simulink model "case4"  (R2024b)
settings: Solver=FixedStepAuto  StartTime=0  StopTime=1  FixedStep=1e-7  RelTol=1e-3
values from neighbouring files (symbols this model uses):
  SG_D_1_D = 0.01056    [IEEE9_case_parameters.m]    (also in case1_parameters.m; case2_parameters.m; case3_parameters.m; case4_parameters.m)
  SG_D_1_EnableSaturation = 0    [IEEE9_case_parameters.m]    (also in case1_parameters.m; case2_parameters.m; case3_parameters.m; case4_parameters.m)
  SG_D_1_f0 = 60    [IEEE9_case_parameters.m]    (also in case1_parameters.m; case2_parameters.m; case3_parameters.m; case4_parameters.m)
  SG_D_1_H = 7.5    [IEEE9_case_parameters.m]    (also in case1_parameters.m; case2_parameters.m; case3_parameters.m; case4_parameters.m)
  SG_D_1_K_A = 20    [IEEE9_case_parameters.m]    (also in case1_parameters.m; case2_parameters.m; case3_parameters.m; case4_parameters.m)
  SG_D_1_K_E = 1.000000e+1    (= 10)    [IEEE9_case_parameters.m]    (also in case1_parameters.m; case2_parameters.m; case3_parameters.m; case4_parameters.m)
  SG_D_1_K_F = 2.363    [IEEE9_case_parameters.m]    (also in case1_parameters.m; case2_parameters.m; case3_parameters.m; case4_parameters.m)
  SG_D_1_K_s = 0.5    [IEEE9_case_parameters.m]    (also in case1_parameters.m = 5; case2_parameters.m = 5; case3_parameters.m = 5; case4_parameters.m = 5)
  SG_D_1_R_a = 0.001088    [IEEE9_case_parameters.m]    (also in case1_parameters.m; case2_parameters.m; case3_parameters.m; case4_parameters.m)
  SG_D_1_S_A = 1    [IEEE9_case_parameters.m]    (also in case1_parameters.m; case2_parameters.m; case3_parameters.m; case4_parameters.m)
  SG_D_1_S_B = 0.103    [IEEE9_case_parameters.m]    (also in case1_parameters.m; case2_parameters.m; case3_parameters.m; case4_parameters.m)
  SG_D_1_S_N = 10.659857    [IEEE9_case_parameters.m]    (also in case1_parameters.m; case2_parameters.m; case3_parameters.m; case4_parameters.m)
  SG_D_1_SpeedPara = 200    [IEEE9_case_parameters.m]    (also in case1_parameters.m; case2_parameters.m; case3_parameters.m; case4_parameters.m)
  SG_D_1_T_0 = 0.720173    [IEEE9_case_parameters.m]    (also in case1_parameters.m = 0.755522; case2_parameters.m = 0.808931; case3_parameters.m = 0.869402; case4_parameters.m = 0.729316)
  SG_D_1_T_1 = 0.3    [IEEE9_case_parameters.m]    (also in case1_parameters.m; case2_parameters.m; case3_parameters.m; case4_parameters.m)
  SG_D_1_T_2 = 0.05    [IEEE9_case_parameters.m]    (also in case1_parameters.m; case2_parameters.m; case3_parameters.m; case4_parameters.m)
  SG_D_1_T_3 = 0.02    [IEEE9_case_parameters.m]    (also in case1_parameters.m; case2_parameters.m; case3_parameters.m; case4_parameters.m)
  SG_D_1_T_4 = 0.005    [IEEE9_case_parameters.m]    (also in case1_parameters.m; case2_parameters.m; case3_parameters.m; case4_parameters.m)
  SG_D_1_T_A = 0.02    [IEEE9_case_parameters.m]    (also in case1_parameters.m; case2_parameters.m; case3_parameters.m; case4_parameters.m)
  SG_D_1_T_dd = 8.000000e+0    (= 8)    [IEEE9_case_parameters.m]    (also in case1_parameters.m; case2_parameters.m; case3_parameters.m; case4_parameters.m)
  SG_D_1_T_ddd = 0.04    [IEEE9_case_parameters.m]    (also in case1_parameters.m; case2_parameters.m; case3_parameters.m; case4_parameters.m)
  SG_D_1_T_E = 0.314    [IEEE9_case_parameters.m]    (also in case1_parameters.m; case2_parameters.m; case3_parameters.m; case4_parameters.m)
  SG_D_1_T_F = 0.35    [IEEE9_case_parameters.m]    (also in case1_parameters.m; case2_parameters.m; case3_parameters.m; case4_parameters.m)
  SG_D_1_T_qd = 0.8    [IEEE9_case_parameters.m]    (also in case1_parameters.m; case2_parameters.m; case3_parameters.m; case4_parameters.m)
  SG_D_1_T_qdd = 0.02    [IEEE9_case_parameters.m]    (also in case1_parameters.m; case2_parameters.m; case3_parameters.m; case4_parameters.m)
  SG_D_1_T_speed = 0.1    [IEEE9_case_parameters.m]    (also in case1_parameters.m = 200; case2_parameters.m = 200; case3_parameters.m = 200; case4_parameters.m = 200)
  SG_D_1_T_w = 0.5    [IEEE9_case_parameters.m]    (also in case1_parameters.m; case2_parameters.m; case3_parameters.m; case4_parameters.m)
  SG_D_1_V_ref = 1.990276    [IEEE9_case_parameters.m]    (also in case1_parameters.m = 2.042296; case2_parameters.m = 2.051388; case3_parameters.m = 2.089584; case4_parameters.m = 2.01845)
  SG_D_1_w_ref = 376.991118    [IEEE9_case_parameters.m]    (also in case1_parameters.m; case2_parameters.m; case3_parameters.m; case4_parameters.m)
  SG_D_1_wb = 6.000000e+1    (= 60)    [IEEE9_case_parameters.m]    (also in case1_parameters.m; case2_parameters.m; case3_parameters.m; case4_parameters.m)
  SG_D_1_x_d = 1.9    [IEEE9_case_parameters.m]    (also in case1_parameters.m; case2_parameters.m; case3_parameters.m; case4_parameters.m)
  SG_D_1_x_dd = 0.302    [IEEE9_case_parameters.m]    (also in case1_parameters.m; case2_parameters.m; case3_parameters.m; case4_parameters.m)
  SG_D_1_x_ddd = 0.204    [IEEE9_case_parameters.m]    (also in case1_parameters.m; case2_parameters.m; case3_parameters.m; case4_parameters.m)
  SG_D_1_x_l = 0.05    [IEEE9_case_parameters.m]    (also in case1_parameters.m; case2_parameters.m; case3_parameters.m; case4_parameters.m)
  SG_D_1_x_q = 1.3    [IEEE9_case_parameters.m]    (also in case1_parameters.m; case2_parameters.m; case3_parameters.m; case4_parameters.m)
  SG_D_1_x_qd = 0.5    [IEEE9_case_parameters.m]    (also in case1_parameters.m; case2_parameters.m; case3_parameters.m; case4_parameters.m)
  SG_D_1_x_qdd = 0.3    [IEEE9_case_parameters.m]    (also in case1_parameters.m; case2_parameters.m; case3_parameters.m; case4_parameters.m)
  SG_D_2_D = 0.02    [IEEE9_case_parameters.m]    (also in case1_parameters.m; case2_parameters.m; case3_parameters.m; case4_parameters.m)
  SG_D_2_EnableSaturation = 0    [IEEE9_case_parameters.m]    (also in case1_parameters.m; case2_parameters.m; case3_parameters.m; case4_parameters.m)
  SG_D_2_f0 = 60    [IEEE9_case_parameters.m]    (also in case1_parameters.m; case2_parameters.m; case3_parameters.m; case4_parameters.m)
  SG_D_2_H = 8.000000e+0    (= 8)    [IEEE9_case_parameters.m]    (also in case1_parameters.m; case2_parameters.m; case3_parameters.m; case4_parameters.m)
  SG_D_2_K_A = 20    [IEEE9_case_parameters.m]    (also in case1_parameters.m; case2_parameters.m; case3_parameters.m; case4_parameters.m)
  SG_D_2_K_E = 1.000000e+1    (= 10)    [IEEE9_case_parameters.m]    (also in case1_parameters.m; case2_parameters.m; case3_parameters.m; case4_parameters.m)
  SG_D_2_K_F = 2.363    [IEEE9_case_parameters.m]    (also in case1_parameters.m; case2_parameters.m; case3_parameters.m; case4_parameters.m)
  SG_D_2_K_s = 0.5    [IEEE9_case_parameters.m]    (also in case1_parameters.m = 4; case2_parameters.m = 4; case3_parameters.m = 4; case4_parameters.m = 4)
  SG_D_2_R_a = 0.001088    [IEEE9_case_parameters.m]    (also in case1_parameters.m; case2_parameters.m; case3_parameters.m; case4_parameters.m)
  SG_D_2_S_A = 1    [IEEE9_case_parameters.m]    (also in case1_parameters.m; case2_parameters.m; case3_parameters.m; case4_parameters.m)
  SG_D_2_S_B = 0.103    [IEEE9_case_parameters.m]    (also in case1_parameters.m; case2_parameters.m; case3_parameters.m; case4_parameters.m)
  SG_D_2_S_N = 10.659857    [IEEE9_case_parameters.m]    (also in case1_parameters.m; case2_parameters.m; case3_parameters.m; case4_parameters.m)
  SG_D_2_SpeedPara = 200    [IEEE9_case_parameters.m]    (also in case1_parameters.m; case2_parameters.m; case3_parameters.m; case4_parameters.m)
  SG_D_2_T_0 = 1.632913    [IEEE9_case_parameters.m]    (also in case1_parameters.m = 1.632925; case2_parameters.m = 1.632915; case3_parameters.m = 1.632914; case4_parameters.m = 1.632927)
  SG_D_2_T_1 = 0.2    [IEEE9_case_parameters.m]    (also in case1_parameters.m; case2_parameters.m; case3_parameters.m; case4_parameters.m)
  SG_D_2_T_2 = 0.05    [IEEE9_case_parameters.m]    (also in case1_parameters.m; case2_parameters.m; case3_parameters.m; case4_parameters.m)
  SG_D_2_T_3 = 0.02    [IEEE9_case_parameters.m]    (also in case1_parameters.m; case2_parameters.m; case3_parameters.m; case4_parameters.m)
  SG_D_2_T_4 = 0.005    [IEEE9_case_parameters.m]    (also in case1_parameters.m; case2_parameters.m; case3_parameters.m; case4_parameters.m)
  SG_D_2_T_A = 0.02    [IEEE9_case_parameters.m]    (also in case1_parameters.m; case2_parameters.m; case3_parameters.m; case4_parameters.m)
  SG_D_2_T_dd = 7.9    [IEEE9_case_parameters.m]    (also in case1_parameters.m; case2_parameters.m; case3_parameters.m; case4_parameters.m)
  SG_D_2_T_ddd = 0.04    [IEEE9_case_parameters.m]    (also in case1_parameters.m; case2_parameters.m; case3_parameters.m; case4_parameters.m)
  SG_D_2_T_E = 0.314    [IEEE9_case_parameters.m]    (also in case1_parameters.m; case2_parameters.m; case3_parameters.m; case4_parameters.m)
  SG_D_2_T_F = 0.35    [IEEE9_case_parameters.m]    (also in case1_parameters.m; case2_parameters.m; case3_parameters.m; case4_parameters.m)
  SG_D_2_T_qd = 0.8    [IEEE9_case_parameters.m]    (also in case1_parameters.m; case2_parameters.m; case3_parameters.m; case4_parameters.m)
  SG_D_2_T_qdd = 0.015    [IEEE9_case_parameters.m]    (also in case1_parameters.m; case2_parameters.m; case3_parameters.m; case4_parameters.m)
  SG_D_2_T_speed = 0.1    [IEEE9_case_parameters.m]    (also in case1_parameters.m = 150; case2_parameters.m = 150; case3_parameters.m = 150; case4_parameters.m = 150)
  SG_D_2_T_w = 0.35    [IEEE9_case_parameters.m]    (also in case1_parameters.m; case2_parameters.m; case3_parameters.m; case4_parameters.m)
  SG_D_2_V_ref = 2.58547    [IEEE9_case_parameters.m]    (also in case1_parameters.m = 2.597896; case2_parameters.m = 2.587136; case3_parameters.m = 2.586042; case4_parameters.m = 2.599679)
  SG_D_2_w_ref = 376.991118    [IEEE9_case_parameters.m]    (also in case1_parameters.m; case2_parameters.m; case3_parameters.m; case4_parameters.m)
  SG_D_2_wb = 6.000000e+1    (= 60)    [IEEE9_case_parameters.m]    (also in case1_parameters.m; case2_parameters.m; case3_parameters.m; case4_parameters.m)
  SG_D_2_x_d = 1.8    [IEEE9_case_parameters.m]    (also in case1_parameters.m; case2_parameters.m; case3_parameters.m; case4_parameters.m)
  SG_D_2_x_dd = 0.302    [IEEE9_case_parameters.m]    (also in case1_parameters.m; case2_parameters.m; case3_parameters.m; case4_parameters.m)
  SG_D_2_x_ddd = 0.204    [IEEE9_case_parameters.m]    (also in case1_parameters.m; case2_parameters.m; case3_parameters.m; case4_parameters.m)
  SG_D_2_x_l = 0.05    [IEEE9_case_parameters.m]    (also in case1_parameters.m; case2_parameters.m; case3_parameters.m; case4_parameters.m)
  SG_D_2_x_q = 1.25    [IEEE9_case_parameters.m]    (also in case1_parameters.m; case2_parameters.m; case3_parameters.m; case4_parameters.m)
  SG_D_2_x_qd = 0.5    [IEEE9_case_parameters.m]    (also in case1_parameters.m; case2_parameters.m; case3_parameters.m; case4_parameters.m)
  SG_D_2_x_qdd = 0.3    [IEEE9_case_parameters.m]    (also in case1_parameters.m; case2_parameters.m; case3_parameters.m; case4_parameters.m)
  SG_D_3_D = 0.02    [IEEE9_case_parameters.m]    (also in case1_parameters.m; case2_parameters.m; case3_parameters.m; case4_parameters.m)
  SG_D_3_EnableSaturation = 0    [IEEE9_case_parameters.m]    (also in case1_parameters.m; case2_parameters.m; case3_parameters.m; case4_parameters.m)
  SG_D_3_f0 = 60    [IEEE9_case_parameters.m]    (also in case1_parameters.m; case2_parameters.m; case3_parameters.m; case4_parameters.m)
  SG_D_3_H = 7.7    [IEEE9_case_parameters.m]    (also in case1_parameters.m; case2_parameters.m; case3_parameters.m; case4_parameters.m)
  SG_D_3_K_A = 20    [IEEE9_case_parameters.m]    (also in case1_parameters.m; case2_parameters.m; case3_parameters.m; case4_parameters.m)
  SG_D_3_K_E = 1.000000e+1    (= 10)    [IEEE9_case_parameters.m]    (also in case1_parameters.m; case2_parameters.m; case3_parameters.m; case4_parameters.m)
  SG_D_3_K_F = 2.363    [IEEE9_case_parameters.m]    (also in case1_parameters.m; case2_parameters.m; case3_parameters.m; case4_parameters.m)
  SG_D_3_K_s = 0.2    [IEEE9_case_parameters.m]    (also in case1_parameters.m = 2; case2_parameters.m = 2; case3_parameters.m = 2; case4_parameters.m = 2)
  SG_D_3_R_a = 0.001088    [IEEE9_case_parameters.m]    (also in case1_parameters.m; case2_parameters.m; case3_parameters.m; case4_parameters.m)
  SG_D_3_S_A = 1    [IEEE9_case_parameters.m]    (also in case1_parameters.m; case2_parameters.m; case3_parameters.m; case4_parameters.m)
  SG_D_3_S_B = 0.103    [IEEE9_case_parameters.m]    (also in case1_parameters.m; case2_parameters.m; case3_parameters.m; case4_parameters.m)
  SG_D_3_S_N = 10.659857    [IEEE9_case_parameters.m]    (also in case1_parameters.m; case2_parameters.m; case3_parameters.m; case4_parameters.m)
  SG_D_3_SpeedPara = 200    [IEEE9_case_parameters.m]    (also in case1_parameters.m; case2_parameters.m; case3_parameters.m; case4_parameters.m)
  SG_D_3_T_0 = 0.850788    [IEEE9_case_parameters.m]    (also in case1_parameters.m = 0.850786; case2_parameters.m = 0.850787; case3_parameters.m; case4_parameters.m = 0.850786)
  SG_D_3_T_1 = 0.2    [IEEE9_case_parameters.m]    (also in case1_parameters.m; case2_parameters.m; case3_parameters.m; case4_parameters.m)
  SG_D_3_T_2 = 0.05    [IEEE9_case_parameters.m]    (also in case1_parameters.m; case2_parameters.m; case3_parameters.m; case4_parameters.m)
  SG_D_3_T_3 = 0.02    [IEEE9_case_parameters.m]    (also in case1_parameters.m; case2_parameters.m; case3_parameters.m; case4_parameters.m)
  SG_D_3_T_4 = 0.005    [IEEE9_case_parameters.m]    (also in case1_parameters.m; case2_parameters.m; case3_parameters.m; case4_parameters.m)
  SG_D_3_T_A = 0.02    [IEEE9_case_parameters.m]    (also in case1_parameters.m; case2_parameters.m; case3_parameters.m; case4_parameters.m)
  SG_D_3_T_dd = 8.1    [IEEE9_case_parameters.m]    (also in case1_parameters.m; case2_parameters.m; case3_parameters.m; case4_parameters.m)
  SG_D_3_T_ddd = 0.04    [IEEE9_case_parameters.m]    (also in case1_parameters.m; case2_parameters.m; case3_parameters.m; case4_parameters.m)
  SG_D_3_T_E = 0.314    [IEEE9_case_parameters.m]    (also in case1_parameters.m; case2_parameters.m; case3_parameters.m; case4_parameters.m)
  SG_D_3_T_F = 0.35    [IEEE9_case_parameters.m]    (also in case1_parameters.m; case2_parameters.m; case3_parameters.m; case4_parameters.m)
  SG_D_3_T_qd = 0.8    [IEEE9_case_parameters.m]    (also in case1_parameters.m; case2_parameters.m; case3_parameters.m; case4_parameters.m)
  SG_D_3_T_qdd = 0.015    [IEEE9_case_parameters.m]    (also in case1_parameters.m; case2_parameters.m; case3_parameters.m; case4_parameters.m)
  SG_D_3_T_speed = 0.1    [IEEE9_case_parameters.m]    (also in case1_parameters.m = 180; case2_parameters.m = 180; case3_parameters.m = 180; case4_parameters.m = 180)
  SG_D_3_T_w = 0.4    [IEEE9_case_parameters.m]    (also in case1_parameters.m; case2_parameters.m; case3_parameters.m; case4_parameters.m)
  SG_D_3_V_ref = 1.892727    [IEEE9_case_parameters.m]    (also in case1_parameters.m = 1.906439; case2_parameters.m = 1.895535; case3_parameters.m = 1.892105; case4_parameters.m = 1.906598)
  SG_D_3_w_ref = 376.991118    [IEEE9_case_parameters.m]    (also in case1_parameters.m; case2_parameters.m; case3_parameters.m; case4_parameters.m)
  SG_D_3_wb = 6.000000e+1    (= 60)    [IEEE9_case_parameters.m]    (also in case1_parameters.m; case2_parameters.m; case3_parameters.m; case4_parameters.m)
  SG_D_3_x_d = 1.85    [IEEE9_case_parameters.m]    (also in case1_parameters.m; case2_parameters.m; case3_parameters.m; case4_parameters.m)
  SG_D_3_x_dd = 0.302    [IEEE9_case_parameters.m]    (also in case1_parameters.m; case2_parameters.m; case3_parameters.m; case4_parameters.m)
  SG_D_3_x_ddd = 0.204    [IEEE9_case_parameters.m]    (also in case1_parameters.m; case2_parameters.m; case3_parameters.m; case4_parameters.m)
  SG_D_3_x_l = 0.05    [IEEE9_case_parameters.m]    (also in case1_parameters.m; case2_parameters.m; case3_parameters.m; case4_parameters.m)
  SG_D_3_x_q = 1.2    [IEEE9_case_parameters.m]    (also in case1_parameters.m; case2_parameters.m; case3_parameters.m; case4_parameters.m)
  SG_D_3_x_qd = 0.5    [IEEE9_case_parameters.m]    (also in case1_parameters.m; case2_parameters.m; case3_parameters.m; case4_parameters.m)
  SG_D_3_x_qdd = 0.3    [IEEE9_case_parameters.m]    (also in case1_parameters.m; case2_parameters.m; case3_parameters.m; case4_parameters.m)
(part 10 of 12)

== system case4/SG_D_3/d_R_f_SG_D_3_block ==
  note: d_R_f_SG_D_3 in case4
      | $-\frac{R_{f,\mathrm{SG},D,3}-\frac{E_{\mathrm{fd},\mathrm{SG},D,3}\,K_{F}}{T_{F}}}{T_{F}}$
      | Automatically generated on 2025-10-31 19:06:53 .
  State_E_fd_SG_D_3_75620 : Inport
  State_R_f_SG_D_3_7757e : Inport  Port=2
  Constant_K_F_23e20 : Constant  Value=K_F
  Constant_T_F_26e23 : Constant  Value=T_F
  Constant_T_F_4e1dc : Constant  Value=T_F
  Divide_62012 : Product  Inputs=*/
  Divide_a3e6f : Product  Inputs=*/
  Product_83b28 : Product
  Subtract_1a0c1 : Sum  Inputs=+-
  Blockout_d_R_f_SG_D_3_a651a : Outport
  wires:
  State_E_fd_SG_D_3_75620/1 -> Product_83b28/1
  Constant_T_F_4e1dc/1 -> Divide_62012/2
  Constant_K_F_23e20/1 -> Product_83b28/2
  Product_83b28/1 -> Divide_62012/1
  Divide_62012/1 -> Subtract_1a0c1/1
  State_R_f_SG_D_3_7757e/1 -> Subtract_1a0c1/2
  Subtract_1a0c1/1 -> Divide_a3e6f/1
  Constant_T_F_26e23/1 -> Divide_a3e6f/2
  Divide_a3e6f/1 -> Blockout_d_R_f_SG_D_3_a651a/1

== system case4/SG_D_3/d_T_m_SG_D_3_block ==
  note: d_T_m_SG_D_3 in case4
      | $-\frac{T_{m,\mathrm{SG},D,3}-T_{0}+\frac{\mathrm{SpeedPara}\,\left(w_{\mathrm{SG},D,3}-w_{\mathrm{ref}}\right)}{2\,f_{0}\,\pi }}{T_{\mathrm{speed}}}$
      | Automatically generated on 2025-10-31 19:06:44 .
  State_w_SG_D_3_1fb5b : Inport
  State_T_m_SG_D_3_64750 : Inport  Port=2
  Add_c46b6 : Sum
  Add_fa378 : Sum
  Constant_-1_1ec3a : Constant  Value=-1
  Constant_2.0_509d8 : Constant  Value=2.0
  Constant_SpeedPara_126f1 : Constant  Value=SpeedPara
  Constant_T_0_22e02 : Constant  Value=T_0
  Constant_T_speed_c5fdf : Constant  Value=T_speed
  Constant_f0_3af54 : Constant  Value=f0
  Constant_pi_23922 : Constant  Value=pi
  Constant_w_ref_47a24 : Constant  Value=w_ref
  Divide_4f7da : Product  Inputs=*/
  Divide_9fe10 : Product  Inputs=*/
  Product_38669 : Product
  Product_82584 : Product
  Product_d6d1b : Product
  Product_e698e : Product
  Subtract_d3f74 : Sum  Inputs=+-
  Blockout_d_T_m_SG_D_3_1d7fb : Outport
  wires:
  Constant_SpeedPara_126f1/1 -> Product_e698e/1
  Constant_-1_1ec3a/1 -> Product_d6d1b/1
  Constant_w_ref_47a24/1 -> Add_fa378/2
  State_w_SG_D_3_1fb5b/1 -> Product_d6d1b/2
  Constant_2.0_509d8/1 -> Product_38669/1
  Product_d6d1b/1 -> Add_fa378/1
  Constant_pi_23922/1 -> Product_38669/2
  Add_fa378/1 -> Product_e698e/2
  Product_38669/1 -> Product_82584/1
  Constant_f0_3af54/1 -> Product_82584/2
  Product_e698e/1 -> Divide_4f7da/1
  Product_82584/1 -> Divide_4f7da/2
  Divide_4f7da/1 -> Add_c46b6/1
  Constant_T_0_22e02/1 -> Add_c46b6/2
  Add_c46b6/1 -> Subtract_d3f74/1
  State_T_m_SG_D_3_64750/1 -> Subtract_d3f74/2
  Subtract_d3f74/1 -> Divide_9fe10/1
  Constant_T_speed_c5fdf/1 -> Divide_9fe10/2
  Divide_9fe10/1 -> Blockout_d_T_m_SG_D_3_1d7fb/1

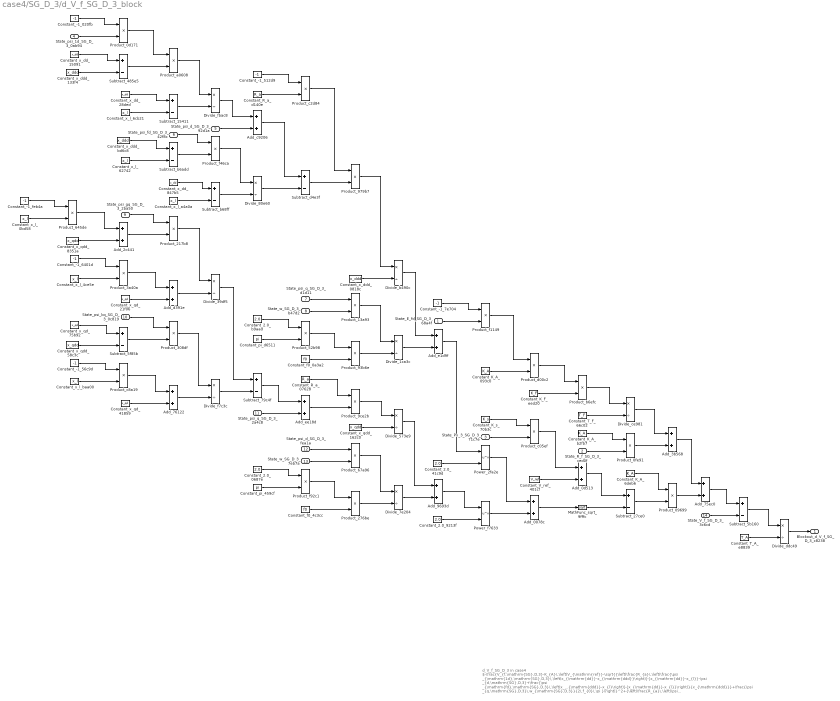
== system case4/SG_D_3/d_V_f_SG_D_3_block ==
  note: d_V_f_SG_D_3 in case4
      | $-\frac{V_{f,\mathrm{SG},D,3}-K_{A}\,\left(V_{\mathrm{ref}}-\sqrt{{\left(\frac{R_{a}\,\left(\frac{\psi _{\mathrm{1d},\mathrm{SG},D,3}\,\left(x_{\mathrm{dd}}-x_{\mathrm{ddd}}\right)}{x_{\mathrm{dd}}-x_{l}}-\psi _{d,\mathrm{SG},D,3}+\frac{\psi _{\mathrm{fd},\mathrm{SG},D,3}\,\left(x_{\mathrm{ddd}}-x_{l}\right)}{x_{\mathrm{dd}}-x_{l}}\right)}{x_{\mathrm{ddd}}}+\frac{\psi _{q,\mathrm{SG},D,3}\,w_{\mathrm{SG},D,3}}{2\,f_{0}\,\pi }\right)}^2+{\left(\frac{R_{a}\,\left(\psi _{q,\mathrm{SG},D,3}+\frac{\psi _{\mathrm{gq},\mathrm{SG},D,3}\,\left(x_{l}-x_{\mathrm{qdd}}\right)}{x_{l}-x_{\mathrm{qd}}}+\frac{\psi _{\mathrm{kq},\mathrm{SG},D,3}\,\left(x_{\mathrm{qd}}-x_{\mathrm{qdd}}\right)}{x_{l}-x_{\mathrm{qd}}}\right)}{x_{\mathrm{qdd}}}+\frac{\psi _{d,\mathrm{SG},D,3}\,w_{\mathrm{SG},D,3}}{2\,f_{0}\,\pi }\right)}^2}+K_{s}\,\mathrm{Px}_{3,\mathrm{SG},D,3}\right)-K_{A}\,R_{f,\mathrm{SG},D,3}+\frac{E_{\mathrm{fd},\mathrm{SG},D,3}\,K_{A}\,K_{F}}{T_{F}}}{T_{A}}$
      | Automatically generated on 2025-10-31 19:06:51 .
  State_E_fd_SG_D_3_68a4f : Inport
  State_R_f_SG_D_3_ced0f : Inport  Port=2
  State_Px_3_SG_D_3_71c7e : Inport  Port=3
  State_psi_1d_SG_D_3_0ab94 : Inport  Port=4
  State_psi_d_SG_D_3_92d1a : Inport  Port=5
  State_psi_fd_SG_D_3_42f8c : Inport  Port=6
  State_psi_q_SG_D_3_d1d11 : Inport  Port=7
  State_w_SG_D_3_b47d2 : Inport  Port=8
  State_psi_gq_SG_D_3_2ba50 : Inport  Port=9
  State_psi_kq_SG_D_3_0c819 : Inport  Port=10
  State_psi_q_SG_D_3_2a4c8 : Inport  Port=11
  State_psi_d_SG_D_3_fea1a : Inport  Port=12
  State_w_SG_D_3_7eb7a : Inport  Port=13
  State_V_f_SG_D_3_3c6cd : Inport  Port=14
  Add_0078c : Sum
  Add_0d513 : Sum
  Add_2c441 : Sum
  Add_3b568 : Sum
  Add_75ec0 : Sum
  Add_76122 : Sum
  Add_9693d : Sum
  Add_c9206 : Sum
  Add_d391e : Sum
  Add_e1d9f : Sum
  Add_ee18d : Sum
  Constant_-1_020fb : Constant  Value=-1
  Constant_-1_512d9 : Constant  Value=-1
  Constant_-1_56c9d : Constant  Value=-1
  Constant_-1_6401d : Constant  Value=-1
  Constant_-1_7e704 : Constant  Value=-1
  Constant_-1_feb4a : Constant  Value=-1
  Constant_2.0_0687e : Constant  Value=2.0
  Constant_2.0_41c9d : Constant  Value=2.0
  Constant_2.0_9213f : Constant  Value=2.0
  Constant_2.0_b9aad : Constant  Value=2.0
  Constant_K_A_093c0 : Constant  Value=K_A
  Constant_K_A_6deb6 : Constant  Value=K_A
  Constant_K_A_b2fb7 : Constant  Value=K_A
  Constant_K_F_eed20 : Constant  Value=K_F
  Constant_K_s_70b3c : Constant  Value=K_s
  Constant_R_a_07628 : Constant  Value=R_a
  Constant_R_a_d140e : Constant  Value=R_a
  Constant_T_A_e8839 : Constant  Value=T_A
  Constant_T_F_66c02 : Constant  Value=T_F
  Constant_V_ref_401cf : Constant  Value=V_ref
  Constant_f0_0a3a2 : Constant  Value=f0
  Constant_f0_4c3cc : Constant  Value=f0
  Constant_pi_459cf : Constant  Value=pi
  Constant_pi_d6511 : Constant  Value=pi
  Constant_x_dd_15091 : Constant  Value=x_dd
  Constant_x_dd_28ded : Constant  Value=x_dd
  Constant_x_dd_847b5 : Constant  Value=x_dd
  Constant_x_ddd_0818c : Constant  Value=x_ddd
  Constant_x_ddd_133f4 : Constant  Value=x_ddd
  Constant_x_ddd_bd6c8 : Constant  Value=x_ddd
  Constant_x_l_0bd58 : Constant  Value=x_l
  Constant_x_l_4ce5e : Constant  Value=x_l
  Constant_x_l_62742 : Constant  Value=x_l
  Constant_x_l_6cb21 : Constant  Value=x_l
  Constant_x_l_a4a0a : Constant  Value=x_l
  Constant_x_l_baa00 : Constant  Value=x_l
  Constant_x_qd_21f06 : Constant  Value=x_qd
  Constant_x_qd_41859 : Constant  Value=x_qd
  Constant_x_qd_75b92 : Constant  Value=x_qd
  Constant_x_qdd_162c0 : Constant  Value=x_qdd
  Constant_x_qdd_58c3c : Constant  Value=x_qdd
  Constant_x_qdd_8351a : Constant  Value=x_qdd
  Divide_1ca3c : Product  Inputs=*/
  Divide_39df5 : Product  Inputs=*/
  Divide_573e9 : Product  Inputs=*/
  Divide_7e204 : Product  Inputs=*/
  Divide_80e60 : Product  Inputs=*/
  Divide_b490c : Product  Inputs=*/
  Divide_ce981 : Product  Inputs=*/
  Divide_ddc49 : Product  Inputs=*/
  Divide_f7c3c : Product  Inputs=*/
  Divide_fbac8 : Product  Inputs=*/
  MathFunc_sqrt_9fffc : Sqrt
  Power_2fa2e : Math  Operator=pow
  Power_f7633 : Math  Operator=pow
  Product_09699 : Product
  Product_0d171 : Product
  Product_0fe91 : Product
  Product_13a93 : Product
  Product_217b8 : Product
  Product_276be : Product
  Product_308df : Product
  Product_3a40a : Product
  Product_52b98 : Product
  Product_645de : Product
  Product_67a96 : Product
  Product_93b6e : Product
  Product_979b7 : Product
  Product_9ce2b : Product
  Product_a0608 : Product
  Product_b6efc : Product
  Product_c05ef : Product
  Product_c2d84 : Product
  Product_c8a19 : Product
  Product_d00c2 : Product
  Product_f1149 : Product
  Product_f46ca : Product
  Product_f92c1 : Product
  Subtract_15411 : Sum  Inputs=+-
  Subtract_27ce0 : Sum  Inputs=+-
  Subtract_485e5 : Sum  Inputs=+-
  Subtract_5b160 : Sum  Inputs=+-
  Subtract_5f85b : Sum  Inputs=+-
  Subtract_79c4f : Sum  Inputs=+-
  Subtract_b68ff : Sum  Inputs=+-
  Subtract_b6add : Sum  Inputs=+-
  Subtract_d4e3f : Sum  Inputs=+-
  Blockout_d_V_f_SG_D_3_c8238 : Outport
  wires:
  Constant_K_A_b2fb7/1 -> Product_0fe91/1
  Constant_-1_feb4a/1 -> Product_645de/1
  Subtract_b6add/1 -> Product_f46ca/2
  Constant_x_l_0bd58/1 -> Product_645de/2
  Divide_7e204/1 -> Add_9693d/2
  Constant_-1_020fb/1 -> Product_0d171/1
  State_psi_1d_SG_D_3_0ab94/1 -> Product_0d171/2
  Constant_x_dd_15091/1 -> Subtract_485e5/1
  Divide_80e60/1 -> Subtract_d4e3f/2
  Product_645de/1 -> Add_2c441/1
  Constant_x_qdd_8351a/1 -> Add_2c441/2
  Constant_x_ddd_133f4/1 -> Subtract_485e5/2
  Constant_2.0_9213f/1 -> Power_f7633/2
  Constant_-1_6401d/1 -> Product_3a40a/1
  Divide_39df5/1 -> Subtract_79c4f/1
  Subtract_15411/1 -> Divide_fbac8/2
  Constant_x_l_4ce5e/1 -> Product_3a40a/2
  Constant_x_qd_75b92/1 -> Subtract_5f85b/1
  State_w_SG_D_3_b47d2/1 -> Product_13a93/2
  Constant_x_qdd_58c3c/1 -> Subtract_5f85b/2
  Constant_2.0_b9aad/1 -> Product_52b98/1
  Constant_-1_56c9d/1 -> Product_c8a19/1
  Constant_pi_d6511/1 -> Product_52b98/2
  Add_c9206/1 -> Subtract_d4e3f/1
  Constant_x_l_baa00/1 -> Product_c8a19/2
  Product_0d171/1 -> Product_a0608/1
  Subtract_485e5/1 -> Product_a0608/2
  Constant_2.0_0687e/1 -> Product_f92c1/1
  Constant_x_dd_28ded/1 -> Subtract_15411/1
  Constant_pi_459cf/1 -> Product_f92c1/2
  Constant_x_l_6cb21/1 -> Subtract_15411/2
  Constant_x_ddd_bd6c8/1 -> Subtract_b6add/1
  Constant_x_l_62742/1 -> Subtract_b6add/2
  State_psi_gq_SG_D_3_2ba50/1 -> Product_217b8/1
  Constant_x_l_a4a0a/1 -> Subtract_b68ff/2
  Add_2c441/1 -> Product_217b8/2
  Product_3a40a/1 -> Add_d391e/1
  Product_217b8/1 -> Divide_39df5/1
  Constant_x_qd_21f06/1 -> Add_d391e/2
  State_psi_kq_SG_D_3_0c819/1 -> Product_308df/1
  State_psi_q_SG_D_3_d1d11/1 -> Product_13a93/1
  Add_e1d9f/1 -> Power_2fa2e/1
  Subtract_5f85b/1 -> Product_308df/2
  Constant_f0_0a3a2/1 -> Product_93b6e/2
  Product_52b98/1 -> Product_93b6e/1
  Constant_x_qd_41859/1 -> Add_76122/2
  Product_c8a19/1 -> Add_76122/1
  Product_a0608/1 -> Divide_fbac8/1
  State_psi_fd_SG_D_3_42f8c/1 -> Product_f46ca/1
  Constant_x_dd_847b5/1 -> Subtract_b68ff/1
  Add_d391e/1 -> Divide_39df5/2
  Add_0078c/1 -> MathFunc_sqrt_9fffc/1
  Product_308df/1 -> Divide_f7c3c/1
  Add_76122/1 -> Divide_f7c3c/2
  Product_c2d84/1 -> Product_979b7/1
  Divide_fbac8/1 -> Add_c9206/1
  Add_0d513/1 -> Subtract_27ce0/1
  State_psi_d_SG_D_3_92d1a/1 -> Add_c9206/2
  Product_f46ca/1 -> Divide_80e60/1
  Subtract_b68ff/1 -> Divide_80e60/2
  MathFunc_sqrt_9fffc/1 -> Subtract_27ce0/2
  Divide_f7c3c/1 -> Subtract_79c4f/2
  Constant_-1_512d9/1 -> Product_c2d84/1
  Constant_R_a_d140e/1 -> Product_c2d84/2
  Subtract_79c4f/1 -> Add_ee18d/1
  State_psi_q_SG_D_3_2a4c8/1 -> Add_ee18d/2
  Subtract_d4e3f/1 -> Product_979b7/2
  Constant_R_a_07628/1 -> Product_9ce2b/1
  Add_ee18d/1 -> Product_9ce2b/2
  State_psi_d_SG_D_3_fea1a/1 -> Product_67a96/1
  State_w_SG_D_3_7eb7a/1 -> Product_67a96/2
  Product_f92c1/1 -> Product_276be/1
  Constant_f0_4c3cc/1 -> Product_276be/2
  Product_979b7/1 -> Divide_b490c/1
  Constant_x_ddd_0818c/1 -> Divide_b490c/2
  Product_13a93/1 -> Divide_1ca3c/1
  Product_93b6e/1 -> Divide_1ca3c/2
  Product_9ce2b/1 -> Divide_573e9/1
  Constant_x_qdd_162c0/1 -> Divide_573e9/2
  Product_67a96/1 -> Divide_7e204/1
  Product_276be/1 -> Divide_7e204/2
  Divide_b490c/1 -> Add_e1d9f/1
  Divide_1ca3c/1 -> Add_e1d9f/2
  Divide_573e9/1 -> Add_9693d/1
  Constant_-1_7e704/1 -> Product_f1149/1
  State_E_fd_SG_D_3_68a4f/1 -> Product_f1149/2
  Constant_2.0_41c9d/1 -> Power_2fa2e/2
  Add_9693d/1 -> Power_f7633/1
  Product_f1149/1 -> Product_d00c2/1
  Constant_K_A_093c0/1 -> Product_d00c2/2
  Constant_K_s_70b3c/1 -> Product_c05ef/1
  State_Px_3_SG_D_3_71c7e/1 -> Product_c05ef/2
  Power_2fa2e/1 -> Add_0078c/1
  Power_f7633/1 -> Add_0078c/2
  Product_d00c2/1 -> Product_b6efc/1
  Constant_K_F_eed20/1 -> Product_b6efc/2
  Product_c05ef/1 -> Add_0d513/1
  Constant_V_ref_401cf/1 -> Add_0d513/2
  Product_b6efc/1 -> Divide_ce981/1
  Constant_T_F_66c02/1 -> Divide_ce981/2
  Add_75ec0/1 -> Subtract_5b160/1
  State_R_f_SG_D_3_ced0f/1 -> Product_0fe91/2
  Divide_ce981/1 -> Add_3b568/1
  Product_0fe91/1 -> Add_3b568/2
  Constant_K_A_6deb6/1 -> Product_09699/1
  Subtract_27ce0/1 -> Product_09699/2
  Add_3b568/1 -> Add_75ec0/1
  Product_09699/1 -> Add_75ec0/2
  State_V_f_SG_D_3_3c6cd/1 -> Subtract_5b160/2
  Subtract_5b160/1 -> Divide_ddc49/1
  Constant_T_A_e8839/1 -> Divide_ddc49/2
  Divide_ddc49/1 -> Blockout_d_V_f_SG_D_3_c8238/1

== system case4/SG_D_3/d_psi_1d_SG_D_3_block ==
  note: d_psi_1d_SG_D_3 in case4
      | $-\frac{\psi _{\mathrm{1d},\mathrm{SG},D,3}-\psi _{\mathrm{fd},\mathrm{SG},D,3}+\frac{\left(x_{\mathrm{dd}}-x_{l}\right)\,\left(\frac{\psi _{\mathrm{1d},\mathrm{SG},D,3}\,\left(x_{\mathrm{dd}}-x_{\mathrm{ddd}}\right)}{x_{\mathrm{dd}}-x_{l}}-\psi _{d,\mathrm{SG},D,3}+\frac{\psi _{\mathrm{fd},\mathrm{SG},D,3}\,\left(x_{\mathrm{ddd}}-x_{l}\right)}{x_{\mathrm{dd}}-x_{l}}\right)}{x_{\mathrm{ddd}}}}{T_{\mathrm{ddd}}}$
      | Automatically generated on 2025-10-31 19:06:28 .
  State_psi_1d_SG_D_3_d1af3 : Inport
  State_psi_fd_SG_D_3_7715d : Inport  Port=2
  State_psi_1d_SG_D_3_363e1 : Inport  Port=3
  State_psi_d_SG_D_3_4396d : Inport  Port=4
  State_psi_fd_SG_D_3_d6b43 : Inport  Port=5
  Add_4bdaa : Sum
  Add_51183 : Sum
  Add_d2586 : Sum
  Constant_-1_6c76e : Constant  Value=-1
  Constant_-1_8655b : Constant  Value=-1
  Constant_T_ddd_407b4 : Constant  Value=T_ddd
  Constant_x_dd_21d62 : Constant  Value=x_dd
  Constant_x_dd_22a31 : Constant  Value=x_dd
  Constant_x_dd_4d5c9 : Constant  Value=x_dd
  Constant_x_dd_f762d : Constant  Value=x_dd
  Constant_x_ddd_0d527 : Constant  Value=x_ddd
  Constant_x_ddd_97c80 : Constant  Value=x_ddd
  Constant_x_ddd_a3944 : Constant  Value=x_ddd
  Constant_x_l_0a31a : Constant  Value=x_l
  Constant_x_l_a4439 : Constant  Value=x_l
  Constant_x_l_a73e9 : Constant  Value=x_l
  Constant_x_l_c2b3a : Constant  Value=x_l
  Divide_4267b : Product  Inputs=*/
  Divide_8791e : Product  Inputs=*/
  Divide_9f8e0 : Product  Inputs=*/
  Divide_b18ce : Product  Inputs=*/
  Product_01604 : Product
  Product_19398 : Product
  Product_5e55a : Product
  Product_77d05 : Product
  Product_a1216 : Product
  Subtract_02a3c : Sum  Inputs=+-
  Subtract_0c2d8 : Sum  Inputs=+-
  Subtract_24927 : Sum  Inputs=+-
  Subtract_c092d : Sum  Inputs=+-
  Subtract_ea4e0 : Sum  Inputs=+-
  Subtract_f9dff : Sum  Inputs=+-
  Blockout_d_psi_1d_SG_D_3_ecab5 : Outport
  wires:
  Divide_b18ce/1 -> Add_51183/1
  Subtract_24927/1 -> Product_19398/2
  Constant_-1_8655b/1 -> Product_5e55a/1
  Constant_x_dd_21d62/1 -> Subtract_c092d/1
  State_psi_1d_SG_D_3_363e1/1 -> Product_5e55a/2
  Product_5e55a/1 -> Product_19398/1
  Constant_x_dd_4d5c9/1 -> Subtract_24927/1
  Constant_x_ddd_0d527/1 -> Subtract_24927/2
  Constant_x_l_0a31a/1 -> Subtract_c092d/2
  Constant_x_ddd_97c80/1 -> Subtract_0c2d8/1
  Divide_9f8e0/1 -> Blockout_d_psi_1d_SG_D_3_ecab5/1
  Constant_x_l_a73e9/1 -> Subtract_0c2d8/2
  Product_19398/1 -> Divide_b18ce/1
  Subtract_c092d/1 -> Divide_b18ce/2
  State_psi_fd_SG_D_3_d6b43/1 -> Product_77d05/1
  Subtract_0c2d8/1 -> Product_77d05/2
  Constant_x_dd_f762d/1 -> Subtract_02a3c/1
  Constant_x_l_c2b3a/1 -> Subtract_02a3c/2
  State_psi_d_SG_D_3_4396d/1 -> Add_51183/2
  Product_77d05/1 -> Divide_8791e/1
  Subtract_02a3c/1 -> Divide_8791e/2
  Constant_x_dd_22a31/1 -> Subtract_f9dff/1
  Constant_x_l_a4439/1 -> Subtract_f9dff/2
  Add_51183/1 -> Subtract_ea4e0/1
  Divide_8791e/1 -> Subtract_ea4e0/2
  Constant_-1_6c76e/1 -> Product_a1216/1
  State_psi_1d_SG_D_3_d1af3/1 -> Product_a1216/2
  State_psi_fd_SG_D_3_7715d/1 -> Add_d2586/2
  Subtract_f9dff/1 -> Product_01604/1
  Subtract_ea4e0/1 -> Product_01604/2
  Product_a1216/1 -> Add_d2586/1
  Product_01604/1 -> Divide_4267b/1
  Constant_x_ddd_a3944/1 -> Divide_4267b/2
  Add_d2586/1 -> Add_4bdaa/1
  Divide_4267b/1 -> Add_4bdaa/2
  Add_4bdaa/1 -> Divide_9f8e0/1
  Constant_T_ddd_407b4/1 -> Divide_9f8e0/2

== system case4/SG_D_3/d_psi_d_SG_D_3_block ==
  note: d_psi_d_SG_D_3 in case4
      | $2\,\pi \,f_{0}\,\left(v_{d,\mathrm{SG},D,3}\,\sin\left(\theta _{\mathrm{SG},D,3}\right)-v_{q,\mathrm{SG},D,3}\,\cos\left(\theta _{\mathrm{SG},D,3}\right)+\frac{R_{a}\,\left(\frac{\psi _{\mathrm{1d},\mathrm{SG},D,3}\,\left(x_{\mathrm{dd}}-x_{\mathrm{ddd}}\right)}{x_{\mathrm{dd}}-x_{l}}-\psi _{d,\mathrm{SG},D,3}+\frac{\psi _{\mathrm{fd},\mathrm{SG},D,3}\,\left(x_{\mathrm{ddd}}-x_{l}\right)}{x_{\mathrm{dd}}-x_{l}}\right)}{x_{\mathrm{ddd}}}+\frac{\psi _{q,\mathrm{SG},D,3}\,w_{\mathrm{SG},D,3}}{2\,f_{0}\,\pi }\right)$
      | Automatically generated on 2025-10-31 19:06:17 .
  State_psi_1d_SG_D_3_58f75 : Inport
  State_psi_d_SG_D_3_f30ef : Inport  Port=2
  State_psi_fd_SG_D_3_ab767 : Inport  Port=3
  Input_v_d_SG_D_3_d5357 : Inport  Port=4
  State_theta_SG_D_3_ca5af : Inport  Port=5
  Input_v_q_SG_D_3_af468 : Inport  Port=6
  State_theta_SG_D_3_ef297 : Inport  Port=7
  State_psi_q_SG_D_3_aa699 : Inport  Port=8
  State_w_SG_D_3_7fa84 : Inport  Port=9
  Add_1684f : Sum
  Add_79258 : Sum
  Constant_-1_c0eb3 : Constant  Value=-1
  Constant_-2.0_46c7c : Constant  Value=-2.0
  Constant_2.0_8ec95 : Constant  Value=2.0
  Constant_R_a_60d6c : Constant  Value=R_a
  Constant_f0_7ff98 : Constant  Value=f0
  Constant_f0_94ff4 : Constant  Value=f0
  Constant_pi_6b123 : Constant  Value=pi
  Constant_pi_96f67 : Constant  Value=pi
  Constant_x_dd_4d035 : Constant  Value=x_dd
  Constant_x_dd_c7b97 : Constant  Value=x_dd
  Constant_x_dd_eca32 : Constant  Value=x_dd
  Constant_x_ddd_1b203 : Constant  Value=x_ddd
  Constant_x_ddd_61a27 : Constant  Value=x_ddd
  Constant_x_ddd_80719 : Constant  Value=x_ddd
  Constant_x_l_6ffb7 : Constant  Value=x_l
  Constant_x_l_96b12 : Constant  Value=x_l
  Constant_x_l_ac7ef : Constant  Value=x_l
  Divide_5b8eb : Product  Inputs=*/
  Divide_9c5d8 : Product  Inputs=*/
  Divide_f130c : Product  Inputs=*/
  Divide_feb83 : Product  Inputs=*/
  MathFunc_cos_d79c3 : Trigonometry  Operator=cos
  MathFunc_sin_eeaf0 : Trigonometry
  Product_243ad : Product
  Product_27e48 : Product
  Product_34485 : Product
  Product_35f29 : Product
  Product_5f5df : Product
  Product_66873 : Product
  Product_697ee : Product
  Product_6e71b : Product
  Product_8d889 : Product
  Product_c6c49 : Product
  Product_c77af : Product
  Product_ebb42 : Product
  Subtract_21d31 : Sum  Inputs=+-
  Subtract_576e4 : Sum  Inputs=+-
  Subtract_80565 : Sum  Inputs=+-
  Subtract_c6b30 : Sum  Inputs=+-
  Subtract_d4aaa : Sum  Inputs=+-
  Subtract_f827f : Sum  Inputs=+-
  Subtract_f873e : Sum  Inputs=+-
  Blockout_d_psi_d_SG_D_3_4bd44 : Outport
  wires:
  Constant_-1_c0eb3/1 -> Product_66873/1
  Constant_2.0_8ec95/1 -> Product_27e48/1
  Constant_x_dd_eca32/1 -> Subtract_576e4/1
  State_psi_1d_SG_D_3_58f75/1 -> Product_66873/2
  Constant_x_dd_c7b97/1 -> Subtract_80565/1
  Constant_pi_96f67/1 -> Product_27e48/2
  Constant_x_ddd_61a27/1 -> Subtract_576e4/2
  Product_66873/1 -> Product_34485/1
  Product_27e48/1 -> Product_697ee/1
  Subtract_576e4/1 -> Product_34485/2
  Constant_-2.0_46c7c/1 -> Product_5f5df/1
  Constant_x_l_96b12/1 -> Subtract_80565/2
  Constant_x_ddd_80719/1 -> Subtract_f827f/1
  Constant_pi_6b123/1 -> Product_5f5df/2
  Constant_x_l_ac7ef/1 -> Subtract_f827f/2
  Product_243ad/1 -> Divide_f130c/1
  Product_34485/1 -> Divide_feb83/1
  Subtract_80565/1 -> Divide_feb83/2
  State_psi_fd_SG_D_3_ab767/1 -> Product_8d889/1
  Subtract_f827f/1 -> Product_8d889/2
  Constant_x_dd_4d035/1 -> Subtract_c6b30/1
  Constant_x_l_6ffb7/1 -> Subtract_c6b30/2
  Divide_f130c/1 -> Subtract_f873e/2
  Divide_feb83/1 -> Add_1684f/1
  Subtract_21d31/1 -> Product_6e71b/2
  State_psi_d_SG_D_3_f30ef/1 -> Add_1684f/2
  Product_8d889/1 -> Divide_9c5d8/1
  Subtract_c6b30/1 -> Divide_9c5d8/2
  Add_1684f/1 -> Subtract_21d31/1
  Divide_9c5d8/1 -> Subtract_21d31/2
  Product_ebb42/1 -> Add_79258/2
  Constant_R_a_60d6c/1 -> Product_6e71b/1
  Product_c77af/1 -> Product_c6c49/1
  State_theta_SG_D_3_ca5af/1 -> MathFunc_sin_eeaf0/1
  Product_6e71b/1 -> Divide_5b8eb/1
  Constant_x_ddd_1b203/1 -> Divide_5b8eb/2
  Input_v_d_SG_D_3_d5357/1 -> Product_35f29/1
  State_w_SG_D_3_7fa84/1 -> Product_243ad/2
  MathFunc_sin_eeaf0/1 -> Product_35f29/2
  State_theta_SG_D_3_ef297/1 -> MathFunc_cos_d79c3/1
  MathFunc_cos_d79c3/1 -> Product_ebb42/2
  Divide_5b8eb/1 -> Subtract_d4aaa/1
  Product_35f29/1 -> Subtract_d4aaa/2
  Input_v_q_SG_D_3_af468/1 -> Product_ebb42/1
  State_psi_q_SG_D_3_aa699/1 -> Product_243ad/1
  Constant_f0_7ff98/1 -> Product_697ee/2
  Subtract_d4aaa/1 -> Add_79258/1
  Product_697ee/1 -> Divide_f130c/2
  Product_5f5df/1 -> Product_c77af/1
  Constant_f0_94ff4/1 -> Product_c77af/2
  Add_79258/1 -> Subtract_f873e/1
  Subtract_f873e/1 -> Product_c6c49/2
  Product_c6c49/1 -> Blockout_d_psi_d_SG_D_3_4bd44/1

== system case4/SG_D_3/d_psi_fd_SG_D_3_block ==
  note: d_psi_fd_SG_D_3 in case4
      | $-\frac{\psi _{\mathrm{fd},\mathrm{SG},D,3}-E_{\mathrm{fd},\mathrm{SG},D,3}+\left(x_{d}-x_{\mathrm{dd}}\right)\,\left(\frac{\frac{\psi _{\mathrm{1d},\mathrm{SG},D,3}\,\left(x_{\mathrm{dd}}-x_{\mathrm{ddd}}\right)}{x_{\mathrm{dd}}-x_{l}}-\psi _{d,\mathrm{SG},D,3}+\frac{\psi _{\mathrm{fd},\mathrm{SG},D,3}\,\left(x_{\mathrm{ddd}}-x_{l}\right)}{x_{\mathrm{dd}}-x_{l}}}{x_{\mathrm{ddd}}}-\frac{\left(x_{\mathrm{dd}}-x_{\mathrm{ddd}}\right)\,\left(\psi _{\mathrm{1d},\mathrm{SG},D,3}-\psi _{\mathrm{fd},\mathrm{SG},D,3}+\frac{\left(x_{\mathrm{dd}}-x_{l}\right)\,\left(\frac{\psi _{\mathrm{1d},\mathrm{SG},D,3}\,\left(x_{\mathrm{dd}}-x_{\mathrm{ddd}}\right)}{x_{\mathrm{dd}}-x_{l}}-\psi _{d,\mathrm{SG},D,3}+\frac{\psi _{\mathrm{fd},\mathrm{SG},D,3}\,\left(x_{\mathrm{ddd}}-x_{l}\right)}{x_{\mathrm{dd}}-x_{l}}\right)}{x_{\mathrm{ddd}}}\right)}{{\left(x_{\mathrm{dd}}-x_{l}\right)}^2}\right)}{T_{\mathrm{dd}}}$
      | Automatically generated on 2025-10-31 19:06:25 .
  State_E_fd_SG_D_3_ed17d : Inport
  State_psi_fd_SG_D_3_58a78 : Inport  Port=2
  State_psi_1d_SG_D_3_83560 : Inport  Port=3
  State_psi_fd_SG_D_3_42dbd : Inport  Port=4
  State_psi_1d_SG_D_3_3b0bc : Inport  Port=5
  State_psi_d_SG_D_3_8f195 : Inport  Port=6
  State_psi_fd_SG_D_3_830e0 : Inport  Port=7
  State_psi_1d_SG_D_3_b04f8 : Inport  Port=8
  State_psi_d_SG_D_3_7086f : Inport  Port=9
  State_psi_fd_SG_D_3_1261a : Inport  Port=10
  Add_1565f : Sum
  Add_a5a47 : Sum
  Constant_-1_73727 : Constant  Value=-1
  Constant_-1_78375 : Constant  Value=-1
  Constant_-1_92e73 : Constant  Value=-1
  Constant_2.0_6c988 : Constant  Value=2.0
  Constant_T_dd_ca17c : Constant  Value=T_dd
  Constant_x_d_f7392 : Constant  Value=x_d
  Constant_x_dd_336c8 : Constant  Value=x_dd
  Constant_x_dd_4367c : Constant  Value=x_dd
  Constant_x_dd_6ec7a : Constant  Value=x_dd
  Constant_x_dd_8a5d6 : Constant  Value=x_dd
  Constant_x_dd_acd8b : Constant  Value=x_dd
  Constant_x_dd_af67d : Constant  Value=x_dd
  Constant_x_dd_d04a8 : Constant  Value=x_dd
  Constant_x_dd_ee1fc : Constant  Value=x_dd
  Constant_x_dd_f350f : Constant  Value=x_dd
  Constant_x_dd_ffccd : Constant  Value=x_dd
  Constant_x_ddd_03a6e : Constant  Value=x_ddd
  Constant_x_ddd_18223 : Constant  Value=x_ddd
  Constant_x_ddd_405b8 : Constant  Value=x_ddd
  Constant_x_ddd_6349b : Constant  Value=x_ddd
  Constant_x_ddd_6764c : Constant  Value=x_ddd
  Constant_x_ddd_7269b : Constant  Value=x_ddd
  Constant_x_ddd_7c859 : Constant  Value=x_ddd
  Constant_x_l_4ab0b : Constant  Value=x_l
  Constant_x_l_6d2b4 : Constant  Value=x_l
  Constant_x_l_71133 : Constant  Value=x_l
  Constant_x_l_79dd6 : Constant  Value=x_l
  Constant_x_l_7d1a0 : Constant  Value=x_l
  Constant_x_l_c0c3d : Constant  Value=x_l
  Constant_x_l_d36a3 : Constant  Value=x_l
  Constant_x_l_fa324 : Constant  Value=x_l
  Divide_08872 : Product  Inputs=*/
  Divide_2622e : Product  Inputs=*/
  Divide_3b756 : Product  Inputs=*/
  Divide_59c79 : Product  Inputs=*/
  Divide_5b6bc : Product  Inputs=*/
  Divide_8771a : Product  Inputs=*/
  Divide_b8e69 : Product  Inputs=*/
  Divide_c1e96 : Product  Inputs=*/
  Power_58ca7 : Math  Operator=pow
  Product_03dce : Product
  Product_1bbee : Product
  Product_32edc : Product
  Product_4bf8f : Product
  Product_4e6c5 : Product
  Product_89ae2 : Product
  Product_a8fa7 : Product
  Product_bedfd : Product
  Product_df1ed : Product
  Product_e92fd : Product
  Subtract_04133 : Sum  Inputs=+-
  Subtract_09d17 : Sum  Inputs=+-
  Subtract_0c217 : Sum  Inputs=+-
  Subtract_1b93b : Sum  Inputs=+-
  Subtract_4b617 : Sum  Inputs=+-
  Subtract_72ebe : Sum  Inputs=+-
  Subtract_72ee8 : Sum  Inputs=+-
  Subtract_747c3 : Sum  Inputs=+-
  Subtract_77a21 : Sum  Inputs=+-
  Subtract_8a8cb : Sum  Inputs=+-
  Subtract_8e76a : Sum  Inputs=+-
  Subtract_95e10 : Sum  Inputs=+-
  Subtract_a01af : Sum  Inputs=+-
  Subtract_a232a : Sum  Inputs=+-
  Subtract_a7d64 : Sum  Inputs=+-
  Subtract_be41d : Sum  Inputs=+-
  Subtract_c88ba : Sum  Inputs=+-
  Subtract_dc920 : Sum  Inputs=+-
  Subtract_f99dc : Sum  Inputs=+-
  Blockout_d_psi_fd_SG_D_3_1d4a8 : Outport
  wires:
  Product_03dce/1 -> Divide_59c79/1
  Constant_-1_92e73/1 -> Product_e92fd/1
  Subtract_a7d64/1 -> Product_bedfd/2
  State_psi_1d_SG_D_3_3b0bc/1 -> Product_e92fd/2
  Constant_x_l_79dd6/1 -> Subtract_a232a/2
  Constant_x_dd_4367c/1 -> Subtract_a7d64/1
  Constant_x_ddd_405b8/1 -> Subtract_a7d64/2
  Product_e92fd/1 -> Product_bedfd/1
  Constant_x_dd_f350f/1 -> Subtract_4b617/1
  Constant_x_l_7d1a0/1 -> Subtract_4b617/2
  Constant_x_ddd_6764c/1 -> Subtract_747c3/2
  Constant_x_ddd_7269b/1 -> Subtract_8e76a/1
  Constant_x_l_4ab0b/1 -> Subtract_8e76a/2
  Product_4bf8f/1 -> Product_1bbee/1
  Product_bedfd/1 -> Divide_b8e69/1
  Subtract_4b617/1 -> Divide_b8e69/2
  State_psi_fd_SG_D_3_830e0/1 -> Product_df1ed/1
  Constant_x_ddd_18223/1 -> Subtract_a232a/1
  Subtract_8e76a/1 -> Product_df1ed/2
  Constant_x_dd_ee1fc/1 -> Subtract_be41d/1
  Constant_-1_78375/1 -> Product_4bf8f/1
  Constant_x_l_d36a3/1 -> Subtract_be41d/2
  Product_1bbee/1 -> Divide_08872/1
  Divide_b8e69/1 -> Add_a5a47/1
  Product_89ae2/1 -> Divide_c1e96/1
  State_psi_d_SG_D_3_8f195/1 -> Add_a5a47/2
  State_psi_fd_SG_D_3_1261a/1 -> Product_89ae2/1
  Product_df1ed/1 -> Divide_2622e/1
  Constant_x_dd_af67d/1 -> Subtract_dc920/1
  Subtract_be41d/1 -> Divide_2622e/2
  Constant_x_l_c0c3d/1 -> Subtract_72ee8/2
  Constant_x_dd_336c8/1 -> Subtract_04133/1
  Subtract_f99dc/1 -> Product_a8fa7/2
  Constant_x_l_71133/1 -> Subtract_04133/2
  Divide_08872/1 -> Add_1565f/1
  Constant_x_ddd_6349b/1 -> Divide_59c79/2
  Add_a5a47/1 -> Subtract_95e10/1
  Divide_2622e/1 -> Subtract_95e10/2
  State_psi_1d_SG_D_3_b04f8/1 -> Product_4bf8f/2
  Constant_x_l_6d2b4/1 -> Subtract_dc920/2
  Constant_x_dd_8a5d6/1 -> Subtract_747c3/1
  Subtract_04133/1 -> Product_03dce/1
  Add_1565f/1 -> Subtract_09d17/1
  Subtract_95e10/1 -> Product_03dce/2
  Subtract_747c3/1 -> Product_1bbee/2
  Constant_x_dd_ffccd/1 -> Subtract_77a21/1
  Constant_x_l_fa324/1 -> Subtract_77a21/2
  Subtract_a232a/1 -> Product_89ae2/2
  Constant_x_dd_6ec7a/1 -> Subtract_f99dc/1
  Constant_x_ddd_03a6e/1 -> Subtract_f99dc/2
  Product_a8fa7/1 -> Product_4e6c5/1
  State_psi_1d_SG_D_3_83560/1 -> Subtract_8a8cb/1
  Subtract_77a21/1 -> Divide_08872/2
  State_psi_fd_SG_D_3_42dbd/1 -> Subtract_8a8cb/2
  Constant_-1_73727/1 -> Product_a8fa7/1
  Subtract_8a8cb/1 -> Subtract_72ebe/1
  Divide_59c79/1 -> Subtract_72ebe/2
  Constant_x_dd_acd8b/1 -> Subtract_72ee8/1
  Divide_c1e96/1 -> Subtract_09d17/2
  State_psi_d_SG_D_3_7086f/1 -> Add_1565f/2
  Subtract_dc920/1 -> Divide_c1e96/2
  Subtract_72ebe/1 -> Product_4e6c5/2
  Subtract_72ee8/1 -> Power_58ca7/1
  Constant_2.0_6c988/1 -> Power_58ca7/2
  Product_4e6c5/1 -> Divide_3b756/1
  Subtract_c88ba/1 -> Product_32edc/2
  Power_58ca7/1 -> Divide_3b756/2
  Subtract_09d17/1 -> Divide_8771a/1
  Constant_x_ddd_7c859/1 -> Divide_8771a/2
  Constant_x_d_f7392/1 -> Subtract_1b93b/1
  Constant_x_dd_d04a8/1 -> Subtract_1b93b/2
  Divide_3b756/1 -> Subtract_c88ba/1
  Divide_8771a/1 -> Subtract_c88ba/2
  State_E_fd_SG_D_3_ed17d/1 -> Subtract_a01af/1
  State_psi_fd_SG_D_3_58a78/1 -> Subtract_a01af/2
  Subtract_1b93b/1 -> Product_32edc/1
  Subtract_a01af/1 -> Subtract_0c217/1
  Product_32edc/1 -> Subtract_0c217/2
  Subtract_0c217/1 -> Divide_5b6bc/1
  Constant_T_dd_ca17c/1 -> Divide_5b6bc/2
  Divide_5b6bc/1 -> Blockout_d_psi_fd_SG_D_3_1d4a8/1
